simulink model "AB_Final_of_MPC_Bandwidth_Result_UnbalancedNew"  (R2022b)
settings: Solver=FixedStepDiscrete  StartTime=0.0  StopTime=Inf  FixedStep=100e-6  RelTol=1e-3  EnableMultiTasking=on
undefined symbols (not defined in the file): C28x, CPU1, CPU2, CurrentBypassValue, DiscIntNeverNeededParam, Down, GPTRIP1SEL, TZ1, Up
libraries: c2802xlib x20, simulink x17, dspstat3 x13, eeGeneralControl x10, c2837xDlib x5, c280xlib x5, PID_Lib x4, c2000lib x1, spsAlphaBetaZerotoabcLib x1
(part 5 of 10)

== system AB_Final_of_MPC_Bandwidth_Result_UnbalancedNew/Subsystem1/VoltageReferenceCalculation ==
  MPCC_f32RGrid : Inport
  MPCC_f32LGrid : Inport  Port=2
  MPCC_f32SamplingPeriod : Inport  Port=3
  MPCC_f32AngularFrequency : Inport  Port=4
  MPCC_f32DGridCurrent : Inport  Port=5
  MPCC_f32QGridCurrent : Inport  Port=6
  MPCC_f32HarmonicDGridCurrent : Inport  Port=7
  MPCC_f32HarmonicQGridCurrent : Inport  Port=8
  MPCC_f32DGridVoltage : Inport  Port=9
  MPCC_f32QGridVoltage : Inport  Port=10
  MPCC_f32DGridCurrentReference : Inport  Port=11
  MPCC_f32HarmonicDGridCurrentReference : Inport  Port=12
  MPCC_f32QGridCurrentReference : Inport  Port=13
  MPCC_f32HarmonicQGridCurrentReference : Inport  Port=14
  MPCC_f32ElectricalAngle : Inport  Port=15
  MPCC_f32DCLinkVoltage : Inport  Port=16
  MPCC_f32HarmonicDGridVoltage : Inport  Port=17
  MPCC_f32HarmonicQGridVoltage : Inport  Port=18
  ElectricalAngleCompensation : Subsystem
  PredictiveTermsCalculation : Subsystem
  VdqVoltageReferenceCalculation : Subsystem
  MPCC_f32DVoltageReference : Outport
  MPCC_f32QVoltageReference : Outport  Port=2
  MPCC_f32ElectricalAngle_K_1 : Outport  Port=3
  MPCC_f32Predictionterm_A : Outport  Port=4
  MPCC_f32Predictionterm_B : Outport  Port=5
  MPCC_f32Predictionterm_C : Outport  Port=6
  wires:
  MPCC_f32RGrid/1 -> PredictiveTermsCalculation/1(MPCC_f32RGrid)
  PredictiveTermsCalculation/1(MPCC_f32Predictionterm_A) -> MPCC_f32Predictionterm_A/1, [MPCC_f32Predictionterm_A]
  PredictiveTermsCalculation/3(MPCC_f32Predictionterm_C) -> [MPCC_f32Predictionterm_C], MPCC_f32Predictionterm_C/1
  [MPCC_f32Predictionterm_A] -> VdqVoltageReferenceCalculation/1(MPCC_f32Predictionterm_A)
  [MPCC_f32Predictionterm_B] -> VdqVoltageReferenceCalculation/2(MPCC_f32Predictionterm_B)
  [MPCC_f32Predictionterm_C] -> VdqVoltageReferenceCalculation/3(MPCC_f32Predictionterm_C)
  MPCC_f32QGridCurrentReference/1 -> VdqVoltageReferenceCalculation/12(MPCC_f32QGridCurrentReference)
  MPCC_f32QGridCurrent/1 -> VdqVoltageReferenceCalculation/5(MPCC_f32QGridCurrent)
  [MPCC_f32SamplingPeriod] -> VdqVoltageReferenceCalculation/15(MPCC_f32SamplingPeriod)
  MPCC_f32DGridCurrent/1 -> VdqVoltageReferenceCalculation/4(MPCC_f32DGridCurrent)
  MPCC_f32HarmonicDGridCurrent/1 -> VdqVoltageReferenceCalculation/6(MPCC_f32HarmonicDGridCurrent)
  MPCC_f32HarmonicDGridCurrentReference/1 -> VdqVoltageReferenceCalculation/11(MPCC_f32HarmonicDGridCurrentReference)
  MPCC_f32HarmonicQGridCurrent/1 -> VdqVoltageReferenceCalculation/7(MPCC_f32HarmonicQGridCurrent)
  MPCC_f32HarmonicQGridCurrentReference/1 -> VdqVoltageReferenceCalculation/13(MPCC_f32HarmonicQGridCurrentReference)
  [MPCC_f32LGrid] -> VdqVoltageReferenceCalculation/14(MPCC_f32LGrid)
  MPCC_f32DGridCurrentReference/1 -> VdqVoltageReferenceCalculation/10(MPCC_f32DGridCurrentReference)
  MPCC_f32QGridVoltage/1 -> VdqVoltageReferenceCalculation/9(MPCC_f32QGridVoltage)
  MPCC_f32DGridVoltage/1 -> VdqVoltageReferenceCalculation/8(MPCC_f32DGridVoltage)
  MPCC_f32LGrid/1 -> [MPCC_f32LGrid]
  MPCC_f32SamplingPeriod/1 -> [MPCC_f32SamplingPeriod]
  [MPCC_f32LGrid] -> PredictiveTermsCalculation/2(MPCC_f32LGrid)
  [MPCC_f32SamplingPeriod] -> PredictiveTermsCalculation/3(MPCC_f32SamplingPeriod)
  VdqVoltageReferenceCalculation/1(MPCC_f32DVoltageReference) -> MPCC_f32DVoltageReference/1
  VdqVoltageReferenceCalculation/2(MPCC_f32QVoltageReference) -> MPCC_f32QVoltageReference/1
  [MPCC_f32SamplingPeriod] -> ElectricalAngleCompensation/1(MPCC_f32SamplingPeriod)
  MPCC_f32ElectricalAngle/1 -> [MPCC_f32ElectricalAngle]
  MPCC_f32AngularFrequency/1 -> [MPCC_f32AngularFrequency]
  [MPCC_f32AngularFrequency] -> ElectricalAngleCompensation/2(MPCC_f32AngularFrequency)
  [MPCC_f32ElectricalAngle] -> ElectricalAngleCompensation/3(MPCC_f32ElectricalAngle)
  ElectricalAngleCompensation/1(MPCC_f32ElectricalAngle_K_1) -> MPCC_f32ElectricalAngle_K_1/1
  [MPCC_f32AngularFrequency] -> PredictiveTermsCalculation/4(MPCC_f32AngularFrequency)
  PredictiveTermsCalculation/2(MPCC_f32Predictionterm_B) -> MPCC_f32Predictionterm_B/1, [MPCC_f32Predictionterm_B]
  MPCC_f32DCLinkVoltage/1 -> VdqVoltageReferenceCalculation/16(MPCC_f32DCLinkVoltage)
  MPCC_f32HarmonicDGridVoltage/1 -> VdqVoltageReferenceCalculation/17(MPCC_f32HarmonicDGridVoltage)
  MPCC_f32HarmonicQGridVoltage/1 -> VdqVoltageReferenceCalculation/18(MPCC_f32HarmonicQGridVoltage)

== system AB_Final_of_MPC_Bandwidth_Result_UnbalancedNew/Subsystem1/dq_abc ==
  theta : Inport
  vd : Inport  Port=2
  vq : Inport  Port=3
  Subsystem6 : Subsystem
  Ia : Outport
  Ib : Outport  Port=2
  Ic : Outport  Port=3
  wires:
  theta/1 -> Subsystem6/3(theta)
  vq/1 -> Subsystem6/2(In2)
  vd/1 -> Subsystem6/1(In1)
  Subsystem6/3(Ic) -> Ic/1
  Subsystem6/2(Ib) -> Ib/1
  Subsystem6/1(Ia) -> Ia/1

== system AB_Final_of_MPC_Bandwidth_Result_UnbalancedNew/Subsystem1/dq_abc1 ==
  theta : Inport
  vd : Inport  Port=2
  vq : Inport  Port=3
  Cast To Single : DataTypeConversion  OutDataTypeStr=single  SaturateOnIntegerOverflow=off  RndMeth=Floor
  Cast To Single1 : DataTypeConversion  OutDataTypeStr=single  SaturateOnIntegerOverflow=off  RndMeth=Floor
  Cast To Single2 : DataTypeConversion  OutDataTypeStr=single  SaturateOnIntegerOverflow=off  RndMeth=Floor
  Subsystem6 : Subsystem
  Ia : Outport
  Ib : Outport  Port=2
  Ic : Outport  Port=3
  wires:
  theta/1 -> Subsystem6/3(theta)
  vq/1 -> Subsystem6/2(In2)
  vd/1 -> Subsystem6/1(In1)
  Subsystem6/3(Ic) -> Cast To Single2/1
  Subsystem6/2(Ib) -> Cast To Single1/1
  Subsystem6/1(Ia) -> Cast To Single/1
  Cast To Single/1 -> Ia/1
  Cast To Single1/1 -> Ib/1
  Cast To Single2/1 -> Ic/1

== system AB_Final_of_MPC_Bandwidth_Result_UnbalancedNew/Subsystem3/LPF ==
  u_k : Inport
  Add : Sum  Inputs=+-
  Add1 : Sum
  Delay : Delay  DelayLength=1
  Gain : Gain  Gain=single(100/1100)
  y_k : Outport
  wires:
  Delay/1 -> Add/2, Add1/2
  Add/1 -> Gain/1
  Gain/1 -> Add1/1
  Add1/1 -> y_k/1, Delay/1
  u_k/1 -> Add/1

== system AB_Final_of_MPC_Bandwidth_Result_UnbalancedNew/Subsystem3/LPF1 ==
  u_k : Inport
  Add : Sum  Inputs=+-
  Add1 : Sum
  Delay : Delay  DelayLength=1
  Gain : Gain  Gain=single(100/1100)
  y_k : Outport
  wires:
  Delay/1 -> Add/2, Add1/2
  Add/1 -> Gain/1
  Gain/1 -> Add1/1
  Add1/1 -> y_k/1, Delay/1
  u_k/1 -> Add/1

== system AB_Final_of_MPC_Bandwidth_Result_UnbalancedNew/Subsystem3/LPF2 ==
  u_k : Inport
  Add : Sum  Inputs=+-
  Add1 : Sum
  Delay : Delay  DelayLength=1
  Gain : Gain  Gain=single(100/1100)
  y_k : Outport
  wires:
  Delay/1 -> Add/2, Add1/2
  Add/1 -> Gain/1
  Gain/1 -> Add1/1
  Add1/1 -> y_k/1, Delay/1
  u_k/1 -> Add/1

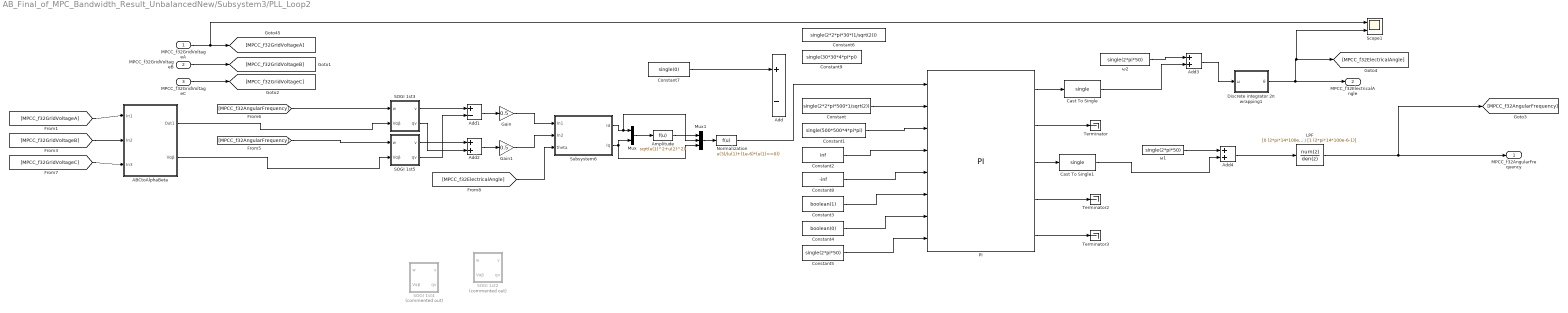
== system AB_Final_of_MPC_Bandwidth_Result_UnbalancedNew/Subsystem3/PLL_Loop2 ==
  MPCC_f32GridVoltageA : Inport
  MPCC_f32GridVoltageB : Inport  Port=2
  MPCC_f32GridVoltageC : Inport  Port=3
  ABCtoAlphaBeta : Subsystem
  Add : Sum  Inputs=+-  OutDataTypeStr=Inherit: Inherit via back propagation
  Add1 : Sum  Inputs=+-
  Add2 : Sum
  Add3 : Sum
  Add4 : Sum
  Amplitude : Fcn  Expr=sqrt(u(1)^2+u(2)^2)
  Cast To Single : DataTypeConversion  OutDataTypeStr=single  SaturateOnIntegerOverflow=off  RndMeth=Floor
  Cast To Single1 : DataTypeConversion  OutDataTypeStr=single  SaturateOnIntegerOverflow=off  RndMeth=Floor
  Constant : Constant  Value=single(2*2*pi*500*1/sqrt(2))  VectorParams1D=off
  Constant1 : Constant  Value=single(500*500*4*pi*pi)
  Constant2 : Constant  Value=inf
  Constant3 : Constant  Value=boolean(1)
  Constant4 : Constant  Value=boolean(0)
  Constant5 : Constant  Value=single(2*pi*50)
  Constant6 : Constant  Value=single(2*2*pi*30*(1/sqrt(2)))
  Constant7 : Constant  Value=single(0)
  Constant8 : Constant  Value=-inf
  Constant9 : Constant  Value=single(30*30*4*pi*pi)
  Discrete integrator 2π wrapping1 : Subsystem
  Gain : Gain  Gain=0.5
  Gain1 : Gain  Gain=0.5
  LPF : DiscreteFilter  Numerator=[0 (2*pi*14*100e-6)]  Denominator=[1 (2*pi*14*100e-6-1)]  InitialStates=50/14/100e-6
  Mux : Mux  Inputs=2
  Mux1 : Mux  Inputs=3
  Normalization : Fcn  Expr=u(3)/(u(1)+(1e-6)*(u(1)==0))
  PI : PID_Lib/PI  SystemSampleTime=-1  VariantActivationTime=update diagram  Latency=0  AutoFrameSizeCalculation=off
  SOGI 1st2 : Subsystem  Commented=on
  SOGI 1st3 : Subsystem
  SOGI 1st4 : Subsystem  Commented=on
  SOGI 1st5 : Subsystem
  Scope1 : Scope  NumInputPorts=2
  Subsystem6 : Subsystem
  Terminator : Terminator
  Terminator2 : Terminator
  Terminator3 : Terminator
  ω1 : Constant  Value=single(2*pi*50)  OutDataTypeStr=single
  ω2 : Constant  Value=single(2*pi*50)  OutDataTypeStr=single
  MPCC_f32AngularFrequency : Outport
  MPCC_f32ElectricalAngle : Outport  Port=2
  wires:
  Constant7/1 -> Add/1
  Constant2/1 -> PI/4
  Constant3/1 -> PI/6
  Constant4/1 -> PI/7
  PI/2 -> Terminator/1
  PI/4 -> Terminator2/1
  PI/5 -> Terminator3/1
  MPCC_f32GridVoltageB/1 -> [MPCC_f32GridVoltageB]
  MPCC_f32GridVoltageC/1 -> [MPCC_f32GridVoltageC]
  Constant8/1 -> PI/5
  PI/1 -> Cast To Single/1
  [MPCC_f32GridVoltageA] -> ABCtoAlphaBeta/1(In1)
  [MPCC_f32GridVoltageB] -> ABCtoAlphaBeta/2(In2)
  [MPCC_f32GridVoltageC] -> ABCtoAlphaBeta/3(In3)
  ABCtoAlphaBeta/2(Vαβ) -> SOGI 1st5/2(Vαβ)
  ABCtoAlphaBeta/1(Out1) -> SOGI 1st3/2(Vαβ)
  SOGI 1st3/1(v) -> Add1/1
  SOGI 1st5/2(qv) -> Add1/2
  SOGI 1st5/1(v) -> Add2/1
  SOGI 1st3/2(qv) -> Add2/2
  Add1/1 -> Gain/1
  Add2/1 -> Gain1/1
  Gain/1 -> Subsystem6/1(In1)
  Gain1/1 -> Subsystem6/2(In2)
  Constant5/1 -> PI/8
  Subsystem6/1(Id) -> Mux1/2, Mux/1
  Subsystem6/2(Iq) -> Mux1/3, Mux/2
  Mux/1 -> Amplitude/1
  Mux1/1 -> Normalization/1
  Amplitude/1 -> Mux1/1
  Cast To Single/1 -> Add3/2
  ω2/1 -> Add3/1
  Add3/1 -> Discrete integrator 2π wrapping1/1(ω)
  Discrete integrator 2π wrapping1/1(θ) -> Scope1/2, [MPCC_f32ElectricalAngle], MPCC_f32ElectricalAngle/1
  PI/3 -> Cast To Single1/1
  ω1/1 -> Add4/1
  Cast To Single1/1 -> Add4/2
  [MPCC_f32ElectricalAngle] -> Subsystem6/3(theta)
  Add4/1 -> LPF/1
  [MPCC_f32AngularFrequency] -> SOGI 1st3/1(w)
  [MPCC_f32AngularFrequency] -> SOGI 1st5/1(w)
  MPCC_f32GridVoltageA/1 -> Scope1/1, [MPCC_f32GridVoltageA]
  Normalization/1 -> PI/1
  Constant/1 -> PI/2
  Constant1/1 -> PI/3
  LPF/1 -> [MPCC_f32AngularFrequency], MPCC_f32AngularFrequency/1

== system AB_Final_of_MPC_Bandwidth_Result_UnbalancedNew/Subsystem3/RateLimiter ==
  Up : Inport
  Ts : Inport  Port=2
  Lo : Inport  Port=3
  U : Inport  Port=4
  Xo : Inport  Port=5
  Rs : Inport  Port=6
  Add1 : Sum  Inputs=+-
  Add2 : Sum
  Data Type Duplicate : DataTypeDuplicate  NumInputPorts=7
  Delay : Delay  DelayLength=1  InitialConditionSource=Input port  ExternalReset=Rising
      settings: InputPortMap=u0,r5,p4
  Product : Product
  Product1 : Product
  Saturation Dynamic : simulink/Discontinuities/Saturation Dynamic  OutMin=[]  OutMax=[]  OutDataTypeStr=Inherit: Same as second input  OutDataType=fixdt(1, 16)  OutScaling=2^-10  DoSatur=off
  Y : Outport
  wires:
  Xo/1 -> Delay/3
  Product1/1 -> Data Type Duplicate/3, Saturation Dynamic/3
  Add1/1 -> Data Type Duplicate/4, Saturation Dynamic/2
  Add2/1 -> Data Type Duplicate/1, Y/1, Delay/1
  Delay/1 -> Data Type Duplicate/2, Add1/2, Add2/2
  U/1 -> Data Type Duplicate/5, Add1/1
  Saturation Dynamic/1 -> Data Type Duplicate/7, Add2/1
  Product/1 -> Data Type Duplicate/6, Saturation Dynamic/1
  Rs/1 -> Delay/2
  Ts/1 -> Product1/1, Product/2
  Lo/1 -> Product1/2
  Up/1 -> Product/1

== system AB_Final_of_MPC_Bandwidth_Result_UnbalancedNew/Subsystem3/RateLimiter1 ==
  Up : Inport
  Ts : Inport  Port=2
  Lo : Inport  Port=3
  U : Inport  Port=4
  Xo : Inport  Port=5
  Rs : Inport  Port=6
  Add1 : Sum  Inputs=+-
  Add2 : Sum
  Data Type Duplicate : DataTypeDuplicate  NumInputPorts=7
  Delay : Delay  DelayLength=1  InitialConditionSource=Input port  ExternalReset=Rising
      settings: InputPortMap=u0,r5,p4
  Product : Product
  Product1 : Product
  Saturation Dynamic : simulink/Discontinuities/Saturation Dynamic  OutMin=[]  OutMax=[]  OutDataTypeStr=Inherit: Same as second input  OutDataType=fixdt(1, 16)  OutScaling=2^-10  DoSatur=off
  Y : Outport
  wires:
  Xo/1 -> Delay/3
  Product1/1 -> Data Type Duplicate/3, Saturation Dynamic/3
  Add1/1 -> Data Type Duplicate/4, Saturation Dynamic/2
  Add2/1 -> Data Type Duplicate/1, Y/1, Delay/1
  Delay/1 -> Data Type Duplicate/2, Add1/2, Add2/2
  U/1 -> Data Type Duplicate/5, Add1/1
  Saturation Dynamic/1 -> Data Type Duplicate/7, Add2/1
  Product/1 -> Data Type Duplicate/6, Saturation Dynamic/1
  Rs/1 -> Delay/2
  Ts/1 -> Product1/1, Product/2
  Lo/1 -> Product1/2
  Up/1 -> Product/1

== system AB_Final_of_MPC_Bandwidth_Result_UnbalancedNew/Subsystem3/RateLimiter2 ==
  Up : Inport
  Ts : Inport  Port=2
  Lo : Inport  Port=3
  U : Inport  Port=4
  Xo : Inport  Port=5
  Rs : Inport  Port=6
  Add1 : Sum  Inputs=+-
  Add2 : Sum
  Data Type Duplicate : DataTypeDuplicate  NumInputPorts=7
  Delay : Delay  DelayLength=1  InitialConditionSource=Input port  ExternalReset=Rising
      settings: InputPortMap=u0,r5,p4
  Product : Product
  Product1 : Product
  Saturation Dynamic : simulink/Discontinuities/Saturation Dynamic  OutMin=[]  OutMax=[]  OutDataTypeStr=Inherit: Same as second input  OutDataType=fixdt(1, 16)  OutScaling=2^-10  DoSatur=off
  Y : Outport
  wires:
  Xo/1 -> Delay/3
  Product1/1 -> Data Type Duplicate/3, Saturation Dynamic/3
  Add1/1 -> Data Type Duplicate/4, Saturation Dynamic/2
  Add2/1 -> Data Type Duplicate/1, Y/1, Delay/1
  Delay/1 -> Data Type Duplicate/2, Add1/2, Add2/2
  U/1 -> Data Type Duplicate/5, Add1/1
  Saturation Dynamic/1 -> Data Type Duplicate/7, Add2/1
  Product/1 -> Data Type Duplicate/6, Saturation Dynamic/1
  Rs/1 -> Delay/2
  Ts/1 -> Product1/1, Product/2
  Lo/1 -> Product1/2
  Up/1 -> Product/1

== system AB_Final_of_MPC_Bandwidth_Result_UnbalancedNew/Subsystem6/Subsystem3 ==
  DiffInput : Inport
  Trigger : Inport  Port=2
  Cast1 : DataTypeConversion  OutDataTypeStr=int8  SaturateOnIntegerOverflow=off  RndMeth=Floor
  Mean1 : dspstat3/Mean  run=on  InputProcessing=Columns as channels (frame based)  reset_popup=Rising edge  directionMode=Each column  dimension=1  roiEnable=off  roiType=Rectangles  roiPortion=Entire ROI  roiOutput=Individual statistics for each ROI  roiFlag=off  roundingMode=Floor  overflowMode=off  outputDataTypeStr=Inherit: Same as accumulator  outputMin=[]  outputMax=[]  outputLastDataTypeStr=Inherit: Same as accumulator
  Mean : Outport
  wires:
  Cast1/1 -> Mean1/2
  DiffInput/1 -> Mean1/1
  Mean1/1 -> Mean/1
  Trigger/1 -> Cast1/1

== system AB_Final_of_MPC_Bandwidth_Result_UnbalancedNew/Subsystem6/Subsystem4 ==
  DiffInput : Inport
  Trigger : Inport  Port=2
  Cast1 : DataTypeConversion  OutDataTypeStr=int8  SaturateOnIntegerOverflow=off  RndMeth=Floor
  Mean1 : dspstat3/Mean  run=on  InputProcessing=Columns as channels (frame based)  reset_popup=Rising edge  directionMode=Each column  dimension=1  roiEnable=off  roiType=Rectangles  roiPortion=Entire ROI  roiOutput=Individual statistics for each ROI  roiFlag=off  roundingMode=Floor  overflowMode=off  outputDataTypeStr=Inherit: Same as accumulator  outputMin=[]  outputMax=[]  outputLastDataTypeStr=Inherit: Same as accumulator
  Mean : Outport
  wires:
  Cast1/1 -> Mean1/2
  DiffInput/1 -> Mean1/1
  Mean1/1 -> Mean/1
  Trigger/1 -> Cast1/1

== system AB_Final_of_MPC_Bandwidth_Result_UnbalancedNew/Subsystem6/Subsystem6 ==
  DiffInput : Inport
  Trigger : Inport  Port=2
  Cast1 : DataTypeConversion  OutDataTypeStr=int8  SaturateOnIntegerOverflow=off  RndMeth=Floor
  Mean1 : dspstat3/Mean  run=on  InputProcessing=Columns as channels (frame based)  reset_popup=Rising edge  directionMode=Each column  dimension=1  roiEnable=off  roiType=Rectangles  roiPortion=Entire ROI  roiOutput=Individual statistics for each ROI  roiFlag=off  roundingMode=Floor  overflowMode=off  outputDataTypeStr=Inherit: Same as accumulator  outputMin=[]  outputMax=[]  outputLastDataTypeStr=Inherit: Same as accumulator
  Mean : Outport
  wires:
  Cast1/1 -> Mean1/2
  DiffInput/1 -> Mean1/1
  Mean1/1 -> Mean/1
  Trigger/1 -> Cast1/1

== system AB_Final_of_MPC_Bandwidth_Result_UnbalancedNew/Voltage_Loop/Subsystem5 ==
  MPCC_f32DCLink : Inport
  Cast To Single1 : DataTypeConversion  OutDataTypeStr=single  SaturateOnIntegerOverflow=off  RndMeth=Floor
  LPF : Subsystem
  MPCC_f32DCLinkFiltered : Outport
  wires:
  LPF/1(y_k) -> Cast To Single1/1
  MPCC_f32DCLink/1 -> LPF/1(u_k)
  Cast To Single1/1 -> MPCC_f32DCLinkFiltered/1  "Iau"

== system AB_Final_of_MPC_Bandwidth_Result_UnbalancedNew/Subsystem1/ABCtoD/LPF ==
  u_k : Inport
  Add : Sum  Inputs=+-
  Add1 : Sum
  Delay : Delay  DelayLength=1
  Gain : Gain  Gain=single(100/(100+200000))
  y_k : Outport
  wires:
  Delay/1 -> Add/2, Add1/2
  Add/1 -> Gain/1
  Gain/1 -> Add1/1
  Add1/1 -> y_k/1, Delay/1
  u_k/1 -> Add/1

== system AB_Final_of_MPC_Bandwidth_Result_UnbalancedNew/Subsystem1/ABCtoD/LPF1 ==
  u_k : Inport
  Add : Sum  Inputs=+-
  Add1 : Sum
  Delay : Delay  DelayLength=1
  Gain : Gain  Gain=single(100/(100+80000))
  y_k : Outport
  wires:
  Delay/1 -> Add/2, Add1/2
  Add/1 -> Gain/1
  Gain/1 -> Add1/1
  Add1/1 -> y_k/1, Delay/1
  u_k/1 -> Add/1

== system AB_Final_of_MPC_Bandwidth_Result_UnbalancedNew/Subsystem1/ABCtoD1Pos/LPF ==
  u_k : Inport
  Add : Sum  Inputs=+-
  Add1 : Sum
  Delay : Delay  DelayLength=1
  Gain : Gain  Gain=single(100/(100+200000))
  y_k : Outport
  wires:
  Delay/1 -> Add/2, Add1/2
  Add/1 -> Gain/1
  Gain/1 -> Add1/1
  Add1/1 -> y_k/1, Delay/1
  u_k/1 -> Add/1

== system AB_Final_of_MPC_Bandwidth_Result_UnbalancedNew/Subsystem1/ABCtoD1Pos/LPF1 ==
  u_k : Inport
  Add : Sum  Inputs=+-
  Add1 : Sum
  Delay : Delay  DelayLength=1
  Gain : Gain  Gain=single(100/(100+80000))
  y_k : Outport
  wires:
  Delay/1 -> Add/2, Add1/2
  Add/1 -> Gain/1
  Gain/1 -> Add1/1
  Add1/1 -> y_k/1, Delay/1
  u_k/1 -> Add/1

== system AB_Final_of_MPC_Bandwidth_Result_UnbalancedNew/Subsystem1/ABCtoD1Pos/LPF2 ==
  u_k : Inport
  Add : Sum  Inputs=+-
  Add1 : Sum
  Delay : Delay  DelayLength=1
  Gain : Gain  Gain=single(100/(100+1000000))
  y_k : Outport
  wires:
  Delay/1 -> Add/2, Add1/2
  Add/1 -> Gain/1
  Gain/1 -> Add1/1
  Add1/1 -> y_k/1, Delay/1
  u_k/1 -> Add/1

== system AB_Final_of_MPC_Bandwidth_Result_UnbalancedNew/Subsystem1/ABCtoD1Pos1/LPF ==
  u_k : Inport
  Add : Sum  Inputs=+-
  Add1 : Sum
  Delay : Delay  DelayLength=1
  Gain : Gain  Gain=single(100/(100+200000))
  y_k : Outport
  wires:
  Delay/1 -> Add/2, Add1/2
  Add/1 -> Gain/1
  Gain/1 -> Add1/1
  Add1/1 -> y_k/1, Delay/1
  u_k/1 -> Add/1

== system AB_Final_of_MPC_Bandwidth_Result_UnbalancedNew/Subsystem1/ABCtoD1Pos1/LPF1 ==
  u_k : Inport
  Add : Sum  Inputs=+-
  Add1 : Sum
  Delay : Delay  DelayLength=1
  Gain : Gain  Gain=single(100/(100+80000))
  y_k : Outport
  wires:
  Delay/1 -> Add/2, Add1/2
  Add/1 -> Gain/1
  Gain/1 -> Add1/1
  Add1/1 -> y_k/1, Delay/1
  u_k/1 -> Add/1

== system AB_Final_of_MPC_Bandwidth_Result_UnbalancedNew/Subsystem1/ABCtoD1Pos1/LPF2 ==
  u_k : Inport
  Add : Sum  Inputs=+-
  Add1 : Sum
  Delay : Delay  DelayLength=1
  Gain : Gain  Gain=single(100/(100+1000000))
  y_k : Outport
  wires:
  Delay/1 -> Add/2, Add1/2
  Add/1 -> Gain/1
  Gain/1 -> Add1/1
  Add1/1 -> y_k/1, Delay/1
  u_k/1 -> Add/1

== system AB_Final_of_MPC_Bandwidth_Result_UnbalancedNew/Subsystem1/ABCtoD1Pos2/LPF ==
  u_k : Inport
  Add : Sum  Inputs=+-
  Add1 : Sum
  Delay : Delay  DelayLength=1
  Gain : Gain  Gain=single(100/(100+200000))
  y_k : Outport
  wires:
  Delay/1 -> Add/2, Add1/2
  Add/1 -> Gain/1
  Gain/1 -> Add1/1
  Add1/1 -> y_k/1, Delay/1
  u_k/1 -> Add/1

== system AB_Final_of_MPC_Bandwidth_Result_UnbalancedNew/Subsystem1/ABCtoD1Pos2/LPF1 ==
  u_k : Inport
  Add : Sum  Inputs=+-
  Add1 : Sum
  Delay : Delay  DelayLength=1
  Gain : Gain  Gain=single(100/(100+80000))
  y_k : Outport
  wires:
  Delay/1 -> Add/2, Add1/2
  Add/1 -> Gain/1
  Gain/1 -> Add1/1
  Add1/1 -> y_k/1, Delay/1
  u_k/1 -> Add/1

== system AB_Final_of_MPC_Bandwidth_Result_UnbalancedNew/Subsystem1/ABCtoD1Pos2/LPF2 ==
  u_k : Inport
  Add : Sum  Inputs=+-
  Add1 : Sum
  Delay : Delay  DelayLength=1
  Gain : Gain  Gain=single(100/(100+1000000))
  y_k : Outport
  wires:
  Delay/1 -> Add/2, Add1/2
  Add/1 -> Gain/1
  Gain/1 -> Add1/1
  Add1/1 -> y_k/1, Delay/1
  u_k/1 -> Add/1

== system AB_Final_of_MPC_Bandwidth_Result_UnbalancedNew/Subsystem1/ABCtoD2/LPF ==
  u_k : Inport
  Add : Sum  Inputs=+-
  Add1 : Sum
  Delay : Delay  DelayLength=1
  Gain : Gain  Gain=single(100/(100+200000))
  y_k : Outport
  wires:
  Delay/1 -> Add/2, Add1/2
  Add/1 -> Gain/1
  Gain/1 -> Add1/1
  Add1/1 -> y_k/1, Delay/1
  u_k/1 -> Add/1

== system AB_Final_of_MPC_Bandwidth_Result_UnbalancedNew/Subsystem1/ABCtoD2/LPF1 ==
  u_k : Inport
  Add : Sum  Inputs=+-
  Add1 : Sum
  Delay : Delay  DelayLength=1
  Gain : Gain  Gain=single(100/(100+80000))
  y_k : Outport
  wires:
  Delay/1 -> Add/2, Add1/2
  Add/1 -> Gain/1
  Gain/1 -> Add1/1
  Add1/1 -> y_k/1, Delay/1
  u_k/1 -> Add/1

== system AB_Final_of_MPC_Bandwidth_Result_UnbalancedNew/Subsystem1/ABCtoD2Neg/LPF ==
  u_k : Inport
  Add : Sum  Inputs=+-
  Add1 : Sum
  Delay : Delay  DelayLength=1
  Gain : Gain  Gain=single(100/(100+200000))
  y_k : Outport
  wires:
  Delay/1 -> Add/2, Add1/2
  Add/1 -> Gain/1
  Gain/1 -> Add1/1
  Add1/1 -> y_k/1, Delay/1
  u_k/1 -> Add/1

== system AB_Final_of_MPC_Bandwidth_Result_UnbalancedNew/Subsystem1/ABCtoD2Neg/LPF1 ==
  u_k : Inport
  Add : Sum  Inputs=+-
  Add1 : Sum
  Delay : Delay  DelayLength=1
  Gain : Gain  Gain=single(100/(100+80000))
  y_k : Outport
  wires:
  Delay/1 -> Add/2, Add1/2
  Add/1 -> Gain/1
  Gain/1 -> Add1/1
  Add1/1 -> y_k/1, Delay/1
  u_k/1 -> Add/1

== system AB_Final_of_MPC_Bandwidth_Result_UnbalancedNew/Subsystem1/ABCtoD2Neg/LPF2 ==
  u_k : Inport
  Add : Sum  Inputs=+-
  Add1 : Sum
  Delay : Delay  DelayLength=1
  Gain : Gain  Gain=single(100/(100+1000000))
  y_k : Outport
  wires:
  Delay/1 -> Add/2, Add1/2
  Add/1 -> Gain/1
  Gain/1 -> Add1/1
  Add1/1 -> y_k/1, Delay/1
  u_k/1 -> Add/1

== system AB_Final_of_MPC_Bandwidth_Result_UnbalancedNew/Subsystem1/ABCtoD2Neg1/LPF ==
  u_k : Inport
  Add : Sum  Inputs=+-
  Add1 : Sum
  Delay : Delay  DelayLength=1
  Gain : Gain  Gain=single(100/(100+200000))
  y_k : Outport
  wires:
  Delay/1 -> Add/2, Add1/2
  Add/1 -> Gain/1
  Gain/1 -> Add1/1
  Add1/1 -> y_k/1, Delay/1
  u_k/1 -> Add/1

== system AB_Final_of_MPC_Bandwidth_Result_UnbalancedNew/Subsystem1/ABCtoD2Neg1/LPF1 ==
  u_k : Inport
  Add : Sum  Inputs=+-
  Add1 : Sum
  Delay : Delay  DelayLength=1
  Gain : Gain  Gain=single(100/(100+80000))
  y_k : Outport
  wires:
  Delay/1 -> Add/2, Add1/2
  Add/1 -> Gain/1
  Gain/1 -> Add1/1
  Add1/1 -> y_k/1, Delay/1
  u_k/1 -> Add/1

== system AB_Final_of_MPC_Bandwidth_Result_UnbalancedNew/Subsystem1/ABCtoD2Neg1/LPF2 ==
  u_k : Inport
  Add : Sum  Inputs=+-
  Add1 : Sum
  Delay : Delay  DelayLength=1
  Gain : Gain  Gain=single(100/(100+1000000))
  y_k : Outport
  wires:
  Delay/1 -> Add/2, Add1/2
  Add/1 -> Gain/1
  Gain/1 -> Add1/1
  Add1/1 -> y_k/1, Delay/1
  u_k/1 -> Add/1

== system AB_Final_of_MPC_Bandwidth_Result_UnbalancedNew/Subsystem1/ABCtoD3/LPF ==
  u_k : Inport
  Add : Sum  Inputs=+-
  Add1 : Sum
  Delay : Delay  DelayLength=1
  Gain : Gain  Gain=single(100/(100+200000))
  y_k : Outport
  wires:
  Delay/1 -> Add/2, Add1/2
  Add/1 -> Gain/1
  Gain/1 -> Add1/1
  Add1/1 -> y_k/1, Delay/1
  u_k/1 -> Add/1

== system AB_Final_of_MPC_Bandwidth_Result_UnbalancedNew/Subsystem1/ABCtoD3/LPF1 ==
  u_k : Inport
  Add : Sum  Inputs=+-
  Add1 : Sum
  Delay : Delay  DelayLength=1
  Gain : Gain  Gain=single(100/(100+80000))
  y_k : Outport
  wires:
  Delay/1 -> Add/2, Add1/2
  Add/1 -> Gain/1
  Gain/1 -> Add1/1
  Add1/1 -> y_k/1, Delay/1
  u_k/1 -> Add/1

== system AB_Final_of_MPC_Bandwidth_Result_UnbalancedNew/Subsystem1/ABCtoDQO/abc_dq ==
  a : Inport
  b : Inport  Port=2
  c : Inport  Port=3
  Subsystem5 : Subsystem
  Id : Outport
  Iq : Outport  Port=2
  wires:
  c/1 -> Subsystem5/3(In3)
  Subsystem5/2(Iq) -> Iq/1
  b/1 -> Subsystem5/2(In2)
  Subsystem5/1(Id) -> Id/1
  a/1 -> Subsystem5/1(In1)

== system AB_Final_of_MPC_Bandwidth_Result_UnbalancedNew/Subsystem1/ABCtoDQO/abc_dq1 ==
  a : Inport
  b : Inport  Port=2
  c : Inport  Port=3
  Subsystem5 : Subsystem
  Id : Outport
  Iq : Outport  Port=2
  wires:
  c/1 -> Subsystem5/3(In3)
  Subsystem5/2(Iq) -> Iq/1
  b/1 -> Subsystem5/2(In2)
  Subsystem5/1(Id) -> Id/1
  a/1 -> Subsystem5/1(In1)

== system AB_Final_of_MPC_Bandwidth_Result_UnbalancedNew/Subsystem1/ABCtoQ/LPF ==
  u_k : Inport
  Add : Sum  Inputs=+-
  Add1 : Sum
  Delay : Delay  DelayLength=1
  Gain : Gain  Gain=single(100/(100+2000000))
  y_k : Outport
  wires:
  Delay/1 -> Add/2, Add1/2
  Add/1 -> Gain/1
  Gain/1 -> Add1/1
  Add1/1 -> y_k/1, Delay/1
  u_k/1 -> Add/1

== system AB_Final_of_MPC_Bandwidth_Result_UnbalancedNew/Subsystem1/ABCtoQ/LPF1 ==
  u_k : Inport
  Add : Sum  Inputs=+-
  Add1 : Sum
  Delay : Delay  DelayLength=1
  Gain : Gain  Gain=single(100/(100+100000))
  y_k : Outport
  wires:
  Delay/1 -> Add/2, Add1/2
  Add/1 -> Gain/1
  Gain/1 -> Add1/1
  Add1/1 -> y_k/1, Delay/1
  u_k/1 -> Add/1

== system AB_Final_of_MPC_Bandwidth_Result_UnbalancedNew/Subsystem1/ABCtoQ/LPF2 ==
  u_k : Inport
  Add : Sum  Inputs=+-
  Add1 : Sum
  Delay : Delay  DelayLength=1
  Gain : Gain  Gain=single(100/(100+1000000))
  y_k : Outport
  wires:
  Delay/1 -> Add/2, Add1/2
  Add/1 -> Gain/1
  Gain/1 -> Add1/1
  Add1/1 -> y_k/1, Delay/1
  u_k/1 -> Add/1

== system AB_Final_of_MPC_Bandwidth_Result_UnbalancedNew/Subsystem1/ABCtoQ/LPF3 ==
  u_k : Inport
  Add : Sum  Inputs=+-
  Add1 : Sum
  Delay : Delay  DelayLength=1
  Gain : Gain  Gain=single(100/(100+80000))
  y_k : Outport
  wires:
  Delay/1 -> Add/2, Add1/2
  Add/1 -> Gain/1
  Gain/1 -> Add1/1
  Add1/1 -> y_k/1, Delay/1
  u_k/1 -> Add/1

== system AB_Final_of_MPC_Bandwidth_Result_UnbalancedNew/Subsystem1/ABCtoQPos1/LPF ==
  u_k : Inport
  Add : Sum  Inputs=+-
  Add1 : Sum
  Delay : Delay  DelayLength=1
  Gain : Gain  Gain=single(100/(100+200000))
  y_k : Outport
  wires:
  Delay/1 -> Add/2, Add1/2
  Add/1 -> Gain/1
  Gain/1 -> Add1/1
  Add1/1 -> y_k/1, Delay/1
  u_k/1 -> Add/1

== system AB_Final_of_MPC_Bandwidth_Result_UnbalancedNew/Subsystem1/ABCtoQPos1/LPF1 ==
  u_k : Inport
  Add : Sum  Inputs=+-
  Add1 : Sum
  Delay : Delay  DelayLength=1
  Gain : Gain  Gain=single(100/(100+80000))
  y_k : Outport
  wires:
  Delay/1 -> Add/2, Add1/2
  Add/1 -> Gain/1
  Gain/1 -> Add1/1
  Add1/1 -> y_k/1, Delay/1
  u_k/1 -> Add/1

== system AB_Final_of_MPC_Bandwidth_Result_UnbalancedNew/Subsystem1/ABCtoQPos1/LPF2 ==
  u_k : Inport
  Add : Sum  Inputs=+-
  Add1 : Sum
  Delay : Delay  DelayLength=1
  Gain : Gain  Gain=single(100/(100+1000000))
  y_k : Outport
  wires:
  Delay/1 -> Add/2, Add1/2
  Add/1 -> Gain/1
  Gain/1 -> Add1/1
  Add1/1 -> y_k/1, Delay/1
  u_k/1 -> Add/1

== system AB_Final_of_MPC_Bandwidth_Result_UnbalancedNew/Subsystem1/AlphaBetaDutiesCalculation/AlphaBetaVoltageReferenceCalculation ==
  MPCC_f32DVoltageReference : Inport
  MPCC_f32QVoltageReference : Inport  Port=2
  MPCC_f32ElectricalAngle_K_1 : Inport  Port=3
  Add : Sum  Inputs=+-
  Add1 : Sum
  Product{,1..3} (4 alike) : Product
  Sin : Trigonometry  Operator=cos
  Sin1 : Trigonometry
  Sin2 : Trigonometry
  Sin3 : Trigonometry  Operator=cos
  MPCC_f32AlphaVoltageReference : Outport
  MPCC_f32BetaVoltageReference : Outport  Port=2
  wires:
  Sin2/1 -> Product2/1
  [MPCC_f32QVoltageReference] -> Product3/2
  Sin1/1 -> Product1/1
  Sin3/1 -> Product3/1
  Product/1 -> Add/1
  [MPCC_f32DVoltageReference] -> Product2/2
  [MPCC_f32ElectricalAngle_K_1] -> Sin2/1
  [MPCC_f32QVoltageReference] -> Product1/2
  Add1/1 -> MPCC_f32BetaVoltageReference/1
  Product2/1 -> Add1/1
  Product3/1 -> Add1/2
  [MPCC_f32ElectricalAngle_K_1] -> Sin3/1
  MPCC_f32DVoltageReference/1 -> [MPCC_f32DVoltageReference]
  Add/1 -> MPCC_f32AlphaVoltageReference/1
  [MPCC_f32ElectricalAngle_K_1] -> Sin/1
  [MPCC_f32DVoltageReference] -> Product/2
  MPCC_f32QVoltageReference/1 -> [MPCC_f32QVoltageReference]
  Product1/1 -> Add/2
  Sin/1 -> Product/1
  [MPCC_f32ElectricalAngle_K_1] -> Sin1/1
  MPCC_f32ElectricalAngle_K_1/1 -> [MPCC_f32ElectricalAngle_K_1]

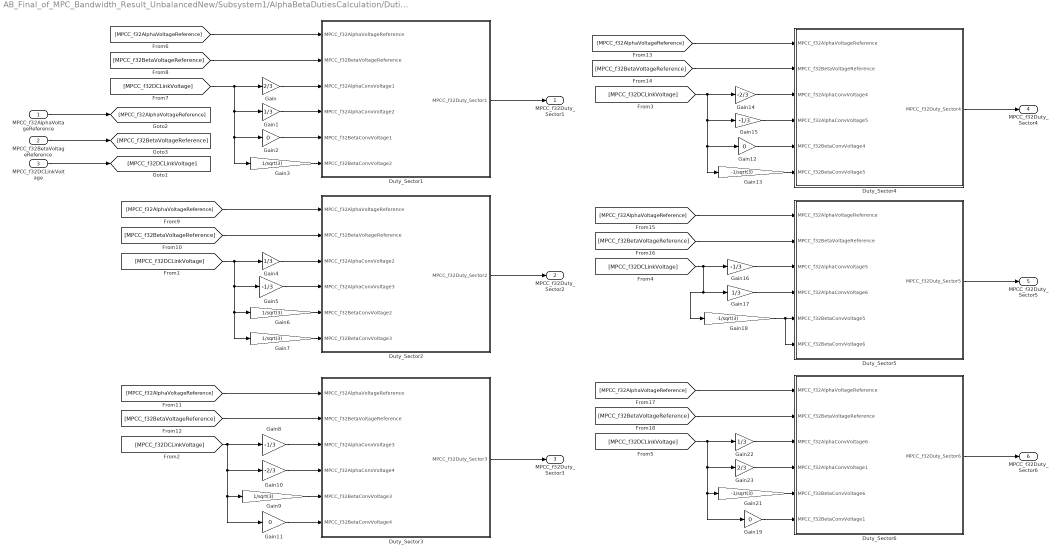
== system AB_Final_of_MPC_Bandwidth_Result_UnbalancedNew/Subsystem1/AlphaBetaDutiesCalculation/DutiesCalculation ==
  MPCC_f32AlphaVoltageReference : Inport
  MPCC_f32BetaVoltageReference : Inport  Port=2
  MPCC_f32DCLinkVoltage : Inport  Port=3
  Duty_Sector1 : Subsystem
  Duty_Sector2 : Subsystem
  Duty_Sector3 : Subsystem
  Duty_Sector4 : Subsystem
  Duty_Sector5 : Subsystem
  Duty_Sector6 : Subsystem
  Gain : Gain  Gain=2/3
  Gain{1,4,17,22} (4 alike) : Gain  Gain=1/3
  Gain10 : Gain  Gain=-2/3
  Gain{2,11..12,19} (4 alike) : Gain  Gain=0
  Gain13 : Gain  Gain=-1/sqrt(3)
  Gain14 : Gain  Gain=-2/3
  Gain{5,8,15..16} (4 alike) : Gain  Gain=-1/3
  Gain18 : Gain  Gain=-1/sqrt(3)
  Gain21 : Gain  Gain=-1/sqrt(3)
  Gain23 : Gain  Gain=2/3
  Gain{3,6..7,9} (4 alike) : Gain  Gain=1/sqrt(3)
  MPCC_f32Duty_Sector1 : Outport
  MPCC_f32Duty_Sector2 : Outport  Port=2
  MPCC_f32Duty_Sector3 : Outport  Port=3
  MPCC_f32Duty_Sector4 : Outport  Port=4
  MPCC_f32Duty_Sector5 : Outport  Port=5
  MPCC_f32Duty_Sector6 : Outport  Port=6
  wires:
  Duty_Sector1/1(MPCC_f32Duty_Sector1) -> MPCC_f32Duty_Sector1/1
  MPCC_f32DCLinkVoltage/1 -> [MPCC_f32DCLinkVoltage]
  Gain/1 -> Duty_Sector1/3(MPCC_f32AlphaConvVoltage1)
  [MPCC_f32DCLinkVoltage] -> Gain2/1, Gain3/1, Gain1/1, Gain/1
  Gain1/1 -> Duty_Sector1/4(MPCC_f32AlphaConvVoltage2)
  Gain2/1 -> Duty_Sector1/5(MPCC_f32BetaConvVoltage1)
  Gain3/1 -> Duty_Sector1/6(MPCC_f32BetaConvVoltage2)
  Duty_Sector2/1(MPCC_f32Duty_Sector2) -> MPCC_f32Duty_Sector2/1
  Gain7/1 -> Duty_Sector2/6(MPCC_f32BetaConvVoltage3)
  Gain4/1 -> Duty_Sector2/3(MPCC_f32AlphaConvVoltage2)
  Gain5/1 -> Duty_Sector2/4(MPCC_f32AlphaConvVoltage3)
  [MPCC_f32DCLinkVoltage] -> Gain6/1, Gain7/1, Gain5/1, Gain4/1
  [MPCC_f32DCLinkVoltage] -> Gain11/1, Gain9/1, Gain10/1, Gain8/1
  Duty_Sector3/1(MPCC_f32Duty_Sector3) -> MPCC_f32Duty_Sector3/1
  Duty_Sector4/1(MPCC_f32Duty_Sector4) -> MPCC_f32Duty_Sector4/1
  Gain13/1 -> Duty_Sector4/6(MPCC_f32BetaConvVoltage5)
  [MPCC_f32DCLinkVoltage] -> Gain12/1, Gain13/1, Gain15/1, Gain14/1
  Duty_Sector5/1(MPCC_f32Duty_Sector5) -> MPCC_f32Duty_Sector5/1
  [MPCC_f32DCLinkVoltage] -> Gain18/1, Gain17/1, Gain16/1
  Duty_Sector6/1(MPCC_f32Duty_Sector6) -> MPCC_f32Duty_Sector6/1
  Gain21/1 -> Duty_Sector6/5(MPCC_f32BetaConvVoltage6)
  [MPCC_f32DCLinkVoltage] -> Gain19/1, Gain21/1, Gain23/1, Gain22/1
  MPCC_f32AlphaVoltageReference/1 -> [MPCC_f32AlphaVoltageReference]
  MPCC_f32BetaVoltageReference/1 -> [MPCC_f32BetaVoltageReference]
  [MPCC_f32AlphaVoltageReference] -> Duty_Sector1/1(MPCC_f32AlphaVoltageReference)
  [MPCC_f32BetaVoltageReference] -> Duty_Sector1/2(MPCC_f32BetaVoltageReference)
  [MPCC_f32AlphaVoltageReference] -> Duty_Sector2/1(MPCC_f32AlphaVoltageReference)
  [MPCC_f32BetaVoltageReference] -> Duty_Sector2/2(MPCC_f32BetaVoltageReference)
  [MPCC_f32AlphaVoltageReference] -> Duty_Sector3/1(MPCC_f32AlphaVoltageReference)
  [MPCC_f32BetaVoltageReference] -> Duty_Sector3/2(MPCC_f32BetaVoltageReference)
  [MPCC_f32AlphaVoltageReference] -> Duty_Sector4/1(MPCC_f32AlphaVoltageReference)
  [MPCC_f32BetaVoltageReference] -> Duty_Sector4/2(MPCC_f32BetaVoltageReference)
  [MPCC_f32AlphaVoltageReference] -> Duty_Sector5/1(MPCC_f32AlphaVoltageReference)
  [MPCC_f32BetaVoltageReference] -> Duty_Sector5/2(MPCC_f32BetaVoltageReference)
  [MPCC_f32AlphaVoltageReference] -> Duty_Sector6/1(MPCC_f32AlphaVoltageReference)
  [MPCC_f32BetaVoltageReference] -> Duty_Sector6/2(MPCC_f32BetaVoltageReference)
  Gain6/1 -> Duty_Sector2/5(MPCC_f32BetaConvVoltage2)
  Gain8/1 -> Duty_Sector3/3(MPCC_f32AlphaConvVoltage3)
  Gain9/1 -> Duty_Sector3/5(MPCC_f32BetaConvVoltage3)
  Gain10/1 -> Duty_Sector3/4(MPCC_f32AlphaConvVoltage4)
  Gain11/1 -> Duty_Sector3/6(MPCC_f32BetaConvVoltage4)
  Gain14/1 -> Duty_Sector4/3(MPCC_f32AlphaConvVoltage4)
  Gain12/1 -> Duty_Sector4/5(MPCC_f32BetaConvVoltage4)
  Gain15/1 -> Duty_Sector4/4(MPCC_f32AlphaConvVoltage5)
  Gain18/1 -> Duty_Sector5/5(MPCC_f32BetaConvVoltage5), Duty_Sector5/6(MPCC_f32BetaConvVoltage6)
  Gain16/1 -> Duty_Sector5/3(MPCC_f32AlphaConvVoltage5)
  Gain17/1 -> Duty_Sector5/4(MPCC_f32AlphaConvVoltage6)
  Gain22/1 -> Duty_Sector6/3(MPCC_f32AlphaConvVoltage6)
  Gain23/1 -> Duty_Sector6/4(MPCC_f32AlphaConvVoltage1)
  Gain19/1 -> Duty_Sector6/6(MPCC_f32BetaConvVoltage1)

== system AB_Final_of_MPC_Bandwidth_Result_UnbalancedNew/Subsystem1/Decoupling_Loop/ABCtoDQOVoltage ==
  PI_f32MDVoltageRef : Inport
  PI_f32MQVoltageRef : Inport  Port=2
  PI_f32MOVoltageRef : Inport  Port=3
  PI_f32ElectricalAngle : Inport  Port=4
  DQOtoA : Subsystem
  DQOtoB : Subsystem
  DQOtoC : Subsystem
  PI_f32MAVoltageRef : Outport
  PI_f32MBVoltageRef : Outport  Port=2
  PI_f32MCVoltageRef : Outport  Port=3
  wires:
  [PI_f32MOVoltageRef] -> DQOtoB/3(PI_f32MOVoltageRef)
  [PI_f32MOVoltageRef] -> DQOtoC/3(PI_f32MOVoltageRef)
  [PI_f32ElectricalAngle] -> DQOtoA/4(PI_f32ElectricalAngle)
  [PI_f32ElectricalAngle] -> DQOtoC/4(PI_f32ElectricalAngle)
  [PI_f32ElectricalAngle] -> DQOtoB/4(PI_f32ElectricalAngle)
  [PI_f32MDVoltageRef] -> DQOtoC/1(PI_f32MDVoltageRef)
  [PI_f32MQVoltageRef] -> DQOtoA/2(PI_f32MQVoltageRef)
  [PI_f32MOVoltageRef] -> DQOtoA/3(PI_f32MOVoltageRef)
  [PI_f32MQVoltageRef] -> DQOtoC/2(PI_f32MQVoltageRef)
  [PI_f32MDVoltageRef] -> DQOtoA/1(PI_f32MDVoltageRef)
  [PI_f32MDVoltageRef] -> DQOtoB/1(PI_f32MDVoltageRef)
  [PI_f32MQVoltageRef] -> DQOtoB/2(PI_f32MQVoltageRef)
  DQOtoA/1(PI_f32MAVoltageRef) -> PI_f32MAVoltageRef/1
  DQOtoB/1(PI_f32MBVoltageRef) -> PI_f32MBVoltageRef/1
  DQOtoC/1(PI_f32MCVoltageRef) -> PI_f32MCVoltageRef/1
  PI_f32MDVoltageRef/1 -> [PI_f32MDVoltageRef]
  PI_f32MQVoltageRef/1 -> [PI_f32MQVoltageRef]
  PI_f32MOVoltageRef/1 -> [PI_f32MOVoltageRef]
  PI_f32ElectricalAngle/1 -> [PI_f32ElectricalAngle]

== system AB_Final_of_MPC_Bandwidth_Result_UnbalancedNew/Subsystem1/Decoupling_Loop/Decoupling_Loop ==
  PI_f32DGridCurrent : Inport
  PI_f32QGridCurrent : Inport  Port=2
  PI_f32DGridVoltage : Inport  Port=3
  PI_f32QGridVoltage : Inport  Port=4
  PI_f32AngularFrequency : Inport  Port=5
  PI_f32DCLinkVoltage : Inport  Port=6
  PI_f32LGrid : Inport  Port=7
  PI_f32DVoltage : Inport  Port=8
  PI_f32QVoltage : Inport  Port=9
  Add : Sum
  Add2 : Sum  OutDataTypeStr=single
  Add3 : Sum
  Add4 : Sum  OutDataTypeStr=single
  Divide : Product  Inputs=*/  OutDataTypeStr=single  RndMeth=Zero  SaturateOnIntegerOverflow=on
  Divide2 : Product  Inputs=*/  OutDataTypeStr=single  RndMeth=Zero  SaturateOnIntegerOverflow=on
  Gain : Gain  Gain=single(-1)
  Gain1 : Gain  Gain=single(2)
  Gain4 : Gain  Gain=single(2)
  Product : Product  Inputs=3
  Product2 : Product  Inputs=3
  PI_f32MDVoltageRef : Outport
  PI_f32MQVoltageRef : Outport  Port=2
  wires:
  [PI_f32DCLinkVoltage] -> Divide/2
  PI_f32DGridCurrent/1 -> [PI_f32DGridCurrent]
  PI_f32QVoltage/1 -> [PI_f32QVoltage]
  PI_f32DGridVoltage/1 -> [PI_f32DGridVoltage]
  [PI_f32QGridCurrent] -> Product/1
  Product/1 -> Gain/1
  PI_f32DVoltage/1 -> [PI_f32DVoltage]
  PI_f32LGrid/1 -> [PI_f32LGrid]
  PI_f32DCLinkVoltage/1 -> [PI_f32DCLinkVoltage]
  [PI_f32AngularFrequency] -> Product/2
  PI_f32AngularFrequency/1 -> [PI_f32AngularFrequency]
  PI_f32QGridCurrent/1 -> [PI_f32QGridCurrent]
  [PI_f32LGrid] -> Product/3
  PI_f32QGridVoltage/1 -> [PI_f32QGridVoltage]
  Add/1 -> Add2/1
  ? -> Add2/2
  Product2/1 -> Add3/1
  [PI_f32DCLinkVoltage] -> Divide2/2
  [PI_f32DGridCurrent] -> Product2/1
  [PI_f32LGrid] -> Product2/3
  ? -> Add4/2
  Add3/1 -> Add4/1
  [PI_f32AngularFrequency] -> Product2/2
  Divide/1 -> PI_f32MDVoltageRef/1
  Divide2/1 -> PI_f32MQVoltageRef/1
  Gain/1 -> Add/1
  [PI_f32QGridVoltage] -> Add3/2
  Gain4/1 -> Divide/1  "Icu"
  Gain1/1 -> Divide2/1  "Icu"
  [PI_f32DGridVoltage] -> Add/2
  [PI_f32QVoltage] -> Gain1/1
  [PI_f32DVoltage] -> Gain4/1

== system AB_Final_of_MPC_Bandwidth_Result_UnbalancedNew/Subsystem1/Decoupling_Loop/dq_abc ==
  theta : Inport
  vd : Inport  Port=2
  vq : Inport  Port=3
  Subsystem6 : Subsystem
  Ia : Outport
  Ib : Outport  Port=2
  Ic : Outport  Port=3
  wires:
  theta/1 -> Subsystem6/3(theta)
  vd/1 -> Subsystem6/1(In1)
  vq/1 -> Subsystem6/2(In2)
  Subsystem6/1(Ia) -> Ia/1
  Subsystem6/2(Ib) -> Ib/1
  Subsystem6/3(Ic) -> Ic/1

== system AB_Final_of_MPC_Bandwidth_Result_UnbalancedNew/Subsystem1/GridCurrentFirstPrediction/PredictedIdGridCurrentCalculation ==
  MPCC_f32Predictionterm_A : Inport
  MPCC_f32Predictionterm_B : Inport  Port=2
  MPCC_f32Predictionterm_C : Inport  Port=3
  MPCC_f32DGridCurrent : Inport  Port=4
  MPCC_f32QGridCurrent : Inport  Port=5
  MPCC_f32DGridVoltage : Inport  Port=6
  MPCC_f32DConvVoltage : Inport  Port=7
  Add : Sum  Inputs=+++-
  Gain : Gain  Gain=0
  Product{,1..2,4} (4 alike) : Product
  MPCC_f32DGridCurrent_K_1 : Outport
  wires:
  Product/1 -> Add/1
  [MPCC_f32QGridCurrent] -> Product1/2
  [MPCC_f32Predictionterm_A] -> Product/1
  Product1/1 -> Gain/1
  [MPCC_f32DGridVoltage] -> Product2/2
  [MPCC_f32DGridCurrent] -> Product/2
  [MPCC_f32Predictionterm_C] -> Product1/1
  [MPCC_f32Predictionterm_B] -> Product2/1
  MPCC_f32Predictionterm_A/1 -> [MPCC_f32Predictionterm_A]
  MPCC_f32Predictionterm_B/1 -> [MPCC_f32Predictionterm_B]
  MPCC_f32Predictionterm_C/1 -> [MPCC_f32Predictionterm_C]
  MPCC_f32DGridCurrent/1 -> [MPCC_f32DGridCurrent]
  MPCC_f32QGridCurrent/1 -> [MPCC_f32QGridCurrent]
  MPCC_f32DGridVoltage/1 -> [MPCC_f32DGridVoltage]
  MPCC_f32DConvVoltage/1 -> [MPCC_f32DConvVoltage]
  Add/1 -> MPCC_f32DGridCurrent_K_1/1
  [MPCC_f32Predictionterm_B] -> Product4/1
  [MPCC_f32DConvVoltage] -> Product4/2
  Product2/1 -> Add/3
  Product4/1 -> Add/4
  Gain/1 -> Add/2

== system AB_Final_of_MPC_Bandwidth_Result_UnbalancedNew/Subsystem1/GridCurrentFirstPrediction/PredictedIqGridCurrentCalculation ==
  MPCC_f32Predictionterm_A : Inport
  MPCC_f32Predictionterm_B : Inport  Port=2
  MPCC_f32Predictionterm_C : Inport  Port=3
  MPCC_f32DGridCurrent : Inport  Port=4
  MPCC_f32QGridCurrent : Inport  Port=5
  MPCC_f32QGridVoltage : Inport  Port=6
  MPCC_f32QConvVoltage : Inport  Port=7
  Add : Sum  Inputs=+-+-
  Gain : Gain  Gain=0
  Product : Product  OutDataTypeStr=Inherit: Inherit via back propagation
  Product1 : Product
  Product2 : Product
  Product4 : Product
  MPCC_f32QVoltageReference : Outport
  wires:
  Product/1 -> Add/1
  [MPCC_f32DGridCurrent] -> Product1/2
  [MPCC_f32Predictionterm_A] -> Product/1
  Product1/1 -> Gain/1
  [MPCC_f32QGridVoltage] -> Product2/2
  [MPCC_f32QGridCurrent] -> Product/2
  [MPCC_f32Predictionterm_C] -> Product1/1
  [MPCC_f32Predictionterm_B] -> Product2/1
  MPCC_f32Predictionterm_A/1 -> [MPCC_f32Predictionterm_A]
  MPCC_f32Predictionterm_B/1 -> [MPCC_f32Predictionterm_B]
  MPCC_f32Predictionterm_C/1 -> [MPCC_f32Predictionterm_C]
  MPCC_f32DGridCurrent/1 -> [MPCC_f32DGridCurrent]
  MPCC_f32QGridCurrent/1 -> [MPCC_f32QGridCurrent]
  MPCC_f32QGridVoltage/1 -> [MPCC_f32QGridVoltage]
  MPCC_f32QConvVoltage/1 -> [MPCC_f32QConvVoltage]
  Add/1 -> MPCC_f32QVoltageReference/1
  [MPCC_f32Predictionterm_B] -> Product4/1
  [MPCC_f32QConvVoltage] -> Product4/2
  Product2/1 -> Add/3
  Product4/1 -> Add/4
  Gain/1 -> Add/2

== system AB_Final_of_MPC_Bandwidth_Result_UnbalancedNew/Subsystem1/GridCurrentSecondPrediction/CostFunctionofSectors ==
  MPCC_f32CostFunction_Voltage1 : Inport
  MPCC_f32CostFunction_Voltage2 : Inport  Port=2
  MPCC_f32CostFunction_Voltage3 : Inport  Port=3
  MPCC_f32CostFunction_Voltage4 : Inport  Port=4
  MPCC_f32CostFunction_Voltage5 : Inport  Port=5
  MPCC_f32CostFunction_Voltage6 : Inport  Port=6
  MPCC_f32Duty_Sector1 : Inport  Port=7
  MPCC_f32Duty_Sector2 : Inport  Port=8
  MPCC_f32Duty_Sector3 : Inport  Port=9
  MPCC_f32Duty_Sector4 : Inport  Port=10
  MPCC_f32Duty_Sector5 : Inport  Port=11
  MPCC_f32Duty_Sector6 : Inport  Port=12
  Duty_Sector1 : Subsystem
  Duty_Sector2 : Subsystem
  Duty_Sector3 : Subsystem
  Duty_Sector4 : Subsystem
  Duty_Sector5 : Subsystem
  Duty_Sector6 : Subsystem
  MPCC_f32CostFunction_Sector1 : Outport
  MPCC_f32CostFunction_Sector2 : Outport  Port=2
  MPCC_f32CostFunction_Sector3 : Outport  Port=3
  MPCC_f32CostFunction_Sector4 : Outport  Port=4
  MPCC_f32CostFunction_Sector5 : Outport  Port=5
  MPCC_f32CostFunction_Sector6 : Outport  Port=6
  wires:
  Duty_Sector1/1(MPCC_f32CostFunction_Sector1) -> MPCC_f32CostFunction_Sector1/1
  [MPCC_f32CostFunction_Voltage1] -> Duty_Sector1/1(MPCC_f32CostFunction_Voltage1)
  [MPCC_f32CostFunction_Voltage2] -> Duty_Sector1/2(MPCC_f32CostFunction_Voltage2)
  [MPCC_f32Duty_Sector1] -> Duty_Sector1/3(MPCC_f32Duty_Sector1)
  MPCC_f32Duty_Sector1/1 -> [MPCC_f32Duty_Sector1]
  MPCC_f32CostFunction_Voltage1/1 -> [MPCC_f32CostFunction_Voltage1]
  MPCC_f32CostFunction_Voltage2/1 -> [MPCC_f32CostFunction_Voltage2]
  MPCC_f32CostFunction_Voltage3/1 -> [MPCC_f32CostFunction_Voltage3]
  MPCC_f32CostFunction_Voltage4/1 -> [MPCC_f32CostFunction_Voltage4]
  MPCC_f32CostFunction_Voltage5/1 -> [MPCC_f32CostFunction_Voltage5]
  MPCC_f32CostFunction_Voltage6/1 -> [MPCC_f32CostFunction_Voltage6]
  MPCC_f32Duty_Sector2/1 -> [MPCC_f32Duty_Sector2]
  MPCC_f32Duty_Sector3/1 -> [MPCC_f32Duty_Sector3]
  MPCC_f32Duty_Sector4/1 -> [MPCC_f32Duty_Sector4]
  MPCC_f32Duty_Sector5/1 -> [MPCC_f32Duty_Sector5]
  MPCC_f32Duty_Sector6/1 -> [MPCC_f32Duty_Sector6]
  Duty_Sector2/1(MPCC_f32CostFunction_Sector2) -> MPCC_f32CostFunction_Sector2/1
  [MPCC_f32Duty_Sector2] -> Duty_Sector2/3(MPCC_f32Duty_Sector2)
  [MPCC_f32CostFunction_Voltage3] -> Duty_Sector2/2(MPCC_f32CostFunction_Voltage3)
  [MPCC_f32CostFunction_Voltage2] -> Duty_Sector2/1(MPCC_f32CostFunction_Voltage2)
  [MPCC_f32CostFunction_Voltage4] -> Duty_Sector3/2(MPCC_f32CostFunction_Voltage4)
  [MPCC_f32CostFunction_Voltage3] -> Duty_Sector3/1(MPCC_f32CostFunction_Voltage3)
  Duty_Sector3/1(MPCC_f32CostFunction_Sector3) -> MPCC_f32CostFunction_Sector3/1
  [MPCC_f32Duty_Sector3] -> Duty_Sector3/3(MPCC_f32Duty_Sector3)
  [MPCC_f32CostFunction_Voltage4] -> Duty_Sector4/1(MPCC_f32CostFunction_Voltage4)
  Duty_Sector4/1(MPCC_f32CostFunction_Sector4) -> MPCC_f32CostFunction_Sector4/1
  [MPCC_f32Duty_Sector4] -> Duty_Sector4/3(MPCC_f32Duty_Sector4)
  [MPCC_f32CostFunction_Voltage5] -> Duty_Sector4/2(MPCC_f32CostFunction_Voltage5)
  [MPCC_f32CostFunction_Voltage5] -> Duty_Sector5/1(MPCC_f32CostFunction_Voltage5)
  [MPCC_f32Duty_Sector5] -> Duty_Sector5/3(MPCC_f32Duty_Sector5)
  Duty_Sector5/1(MPCC_f32CostFunction_Sector5) -> MPCC_f32CostFunction_Sector5/1
  [MPCC_f32CostFunction_Voltage6] -> Duty_Sector5/2(MPCC_f32CostFunction_Voltage6)
  [MPCC_f32CostFunction_Voltage1] -> Duty_Sector6/2(MPCC_f32CostFunction_Voltage1)
  [MPCC_f32Duty_Sector6] -> Duty_Sector6/3(MPCC_f32Duty_Sector6)
  Duty_Sector6/1(MPCC_f32CostFunction_Sector6) -> MPCC_f32CostFunction_Sector6/1
  [MPCC_f32CostFunction_Voltage6] -> Duty_Sector6/1(MPCC_f32CostFunction_Voltage6)
